simulink model "virtual_world_without_car"  (R2015b)
settings: Solver=ode3  StartTime=5  StopTime=simulationStop  FixedStep=0.04  RelTol=1e-3
PostLoadFcn:
  | if ~exist('visionlib','file') sl3ddemo_callbacks('DelayedError', gcs, 'Missing Library', 'This example requires Computer Vision System Toolbox.'); end; load octavia_testlap
values from neighbouring files (symbols this model uses):
  rotation_matrix = R_z * R_y * R_x    [frames_acquisition.m]
  sampleTime = 0.04    [frames_acquisition.m]
libraries: vrlib x26, visionsinks x1
Description:
  | Vehicle Dynamics Visualization with Video Output
  | 
  | This model extends the vr_octavia example and shows how to use
  | video output from the VR Video Output block.
  | 
  | This model performs a few simple operations on the output video signal.
  | The Video Viewer display then shows the resulting video stream where
  | the image edges are detected.
  | 
  | This model requires the Computer Vision System Toolbox(TM) product.
  | 
  | Such model has been used to implement an educational platform for
  | simulating Unmanned Aerial Vehicles aimed to detect and track moving
  | objects
settings Model: ExtModeArmWhenConnect=off  Creator=Giuseppe Silano  LastModifiedBy=giuse
settings DataIOCC: SaveFormat=Array  SignalLoggingName=sigsOut
settings OptimizationCC: BooleanDataType=off  OptimizeBlockIOStorage=off  BufferReuse=off  GlobalBufferReuse=off  ExpressionFolding=off  ExpressionDepthLimit=2147483647  LocalBlockOutputs=off  InitFltsAndDblsToZero=on
settings DebuggingCC: UnderspecifiedInitializationDetection=Classic  MergeDetectMultiDrivingBlocksExec=none  CheckExecutionContextPreStartOutputMsg=on  CheckExecutionContextRuntimeOutputMsg=on  SignalResolutionControl=TryResolveAllWithWarning  MultiTaskDSMMsg=warning  MultiTaskCondExecSysMsg=none  FcnCallInpInsideContextMsg=UseLocalSettings  StateNameClashWarn=warning
settings HardwareCC: ProdBitPerPointer=32  ProdLargestAtomicFloat=None  ProdIntDivRoundTo=Undefined  ProdEndianess=Unspecified  ProdWordSize=32  ProdHWDeviceType=32-bit Generic
settings RTWCC: RetainRTWFile=on
settings GRTTargetCC: TargetFcnLib=ansi_tfl_tmw.mat  GeneratePreprocessorConditionals=Disable all  CombineOutputUpdateFcns=off  GRTInterface=on
settings ConfigComp: CovModelRefEnable=Off  CovSFcnEnable=off

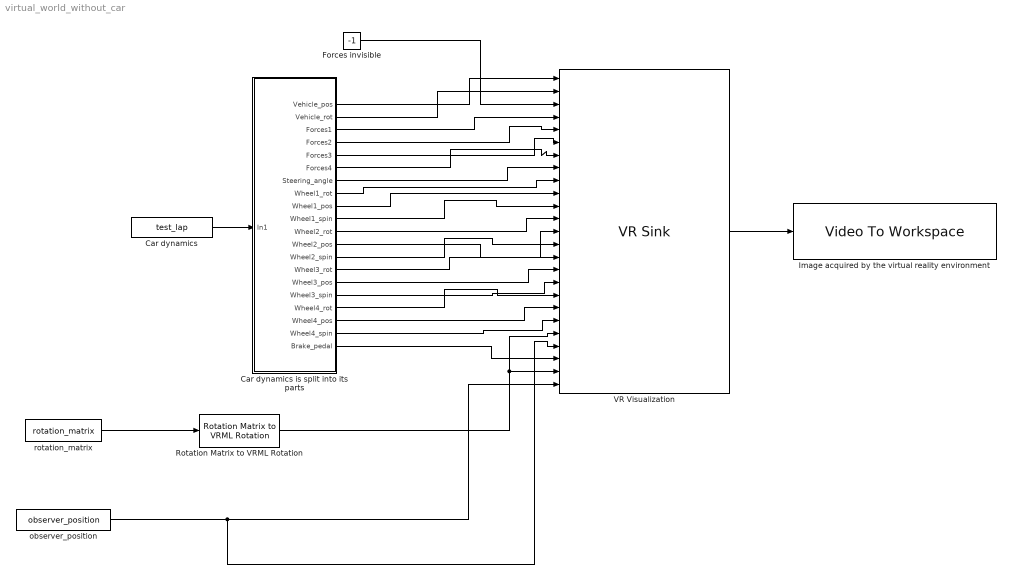
== system virtual_world_without_car ==
  Car dynamics : FromWorkspace  VariableName=test_lap  SampleTime=0.04  OutputAfterFinalValue=Holding final value
  "Car dynamics is split into its parts " : Subsystem
  Forces invisible : Constant  Value=-1
  Image acquired by the virtual reality environment : visionsinks/Video To Workspace  VariableName=image  NumInputs=1  DataLimit=1  DecimationFactor=1  LogFi=off  InPortLabels=R|G|B
  Rotation Matrix to VRML Rotation : vrlib/Utilities/Rotation Matrix to VRML Rotation  maxzero=1e-12
  VR Visualization : vrlib/VR Sink  InstantiateOnLoad=on  SampleTime=sampleTime  ViewEnable=on  RemoteChange=off  RemoteView=on  FieldsWritten=Vehicle_pos_Car1.translation.3.1.1.double#Vehicle_rot_Car1.rotation.4.1.1.double#Forces_visible_Car1.whichChoice.1.1.1.double#Force1_Car1.scale.3.1.1.double#Force2_Car1.scale.3.1.1.double#Force3_Car1.scale.3.1.1.double#Force4_Car1.scale.3.1.1.double#SteeringWheelAngle1_Car1.rotation.4.1.1.double#WheelFL_Car1.rotation.4.1.1.double#WheelFL_Car1.translation.3.1.1.double#WheelSpinFL_Car1.rotation.4.1.1.double#WheelFR_Car1.rotation.4.1.1.double#WheelFR_Car1.translation.3.1.1.double#WheelSpinFR_Car1.rotation.4.1.1.double#WheelRL_Car1.rotation.4.1.1.double#WheelRL_Car1.translation.3.1.1.double#WheelSpinRL_Car1.rotation.4.1.1.double#WheelRR_Car1.rotation.4.1.1.double#WheelRR_Car1.translation.3.1.1.double#WheelSpinRR_Car1.rotation.4.1.1.double#FlyingCamera.orientation.4.1.1.double#FlyingCamera.position.3.1.1.double#Brake_Switch_Car1.whichChoice.1.1.1.double#Osservatore_esterno:drone.orientation.4.1.1.double#Osservatore_esterno:drone.position.3.1.1.double  WorldFileName=octavia_scene.wrl  WorldDescription=Vehicle dynamics visualization  AutoView=on  VideoDimensions=[800 600]  AllowVariableSize=off  FigureProperties="{'Position', 'Name', 'Viewpoint', 'CameraBound', 'CameraDirection', 'CameraPosition', 'CameraUpVector', 'ZoomFactor', 'Antialiasing', 'Headlight', 'Lighting', 'NavPanel', 'Sound', 'StatusBar', 'Stereo3D', 'Stereo3DCameraOffset', 'Stereo3DHIT', 'ToolBar', 'Textures', 'Transparency', 'Triad', 'Wireframe', 'NavZones', 'NavMode', 'NavSpeed', 'CaptureFileFormat', 'CaptureFileName', 'Record2DCompressMethod', 'Record2DCompressQuality', 'Record2D', 'Record2DFileName', 'Record2DFPS'; [5.0000000000000000e+00   9.2000000000000000e+01   5.7600000000000000e+02   3.8000000000000000e+02], 'Vehicle dynamics visualization', 'Car - View from Right Above Ahead', 'on', [0.0000000000000000e+00   0.0000000000000000e+00  -1.0000000000000000e+00], [0.0000000000000000e+00   0.0000000000000000e+00   0.0000000000000000e+00], [0.0000000000000000e+00   1.0000000000000000e+00   0.0000000000000000e+00], [1.0000000000000000e+00], 'on', 'off', 'on', 'halfbar', 'on', 'on', 'off', [1.0000000149011612e-01], [0.0000000000000000e+00], 'on', 'on', 'on', 'none', 'off', 'off', 'walk', 'normal', 'tif', '%f_anim_%n.tif', 'auto', [7.5000000000000000e+01], 'off', '%f_anim_%n.avi', 'auto'; [5.8600000000000000e+02   6.0000000000000000e+01   6.0000000000000000e+02   8.0000000000000000e+02], 'Vehicle dynamics visualization', 'Osservatore_esterno:drone', 'on', [0.0000000000000000e+00   0.0000000000000000e+00  -1.0000000000000000e+00], [0.0000000000000000e+00   0.0000000000000000e+00   0.0000000000000000e+00], [0.0000000000000000e+00   1.0000000000000000e+00   0.0000000000000000e+00], [1.0000000000000000e+00], 'on', 'off', 'on', 'none', 'on', 'off', 'off', [1.0000000149011612e-01], [0.0000000000000000e+00], 'off', 'on', 'on', 'none', 'off', 'off', 'walk', 'normal', 'tif', '%f_anim_%n.tif', 'auto', [7.5000000000000000e+01], 'off', '***video***', [1.5000000000000000e+01]}"
  observer_position : FromWorkspace  VariableName=observer_position  SampleTime=0
  rotation_matrix : Constant  Value=rotation_matrix
  wires:
  Car dynamics/1 -> "Car dynamics is split into its parts "/1(In1)
  VR Visualization/1 -> Image acquired by the virtual reality environment/1
  "Car dynamics is split into its parts "/1(Vehicle_pos) -> VR Visualization/1
  "Car dynamics is split into its parts "/2(Vehicle_rot) -> VR Visualization/2
  Forces invisible/1 -> VR Visualization/3
  "Car dynamics is split into its parts "/3(Forces1) -> VR Visualization/4
  "Car dynamics is split into its parts "/4(Forces2) -> VR Visualization/5
  "Car dynamics is split into its parts "/5(Forces3) -> VR Visualization/6
  "Car dynamics is split into its parts "/6(Forces4) -> VR Visualization/7
  "Car dynamics is split into its parts "/7(Steering_angle) -> VR Visualization/8
  "Car dynamics is split into its parts "/8(Wheel1_rot) -> VR Visualization/9
  "Car dynamics is split into its parts "/9(Wheel1_pos) -> VR Visualization/10
  "Car dynamics is split into its parts "/10(Wheel1_spin) -> VR Visualization/11
  "Car dynamics is split into its parts "/11(Wheel2_rot) -> VR Visualization/12
  "Car dynamics is split into its parts "/12(Wheel2_pos) -> VR Visualization/13
  "Car dynamics is split into its parts "/13(Wheel2_spin) -> VR Visualization/14
  "Car dynamics is split into its parts "/14(Wheel3_rot) -> VR Visualization/15
  "Car dynamics is split into its parts "/15(Wheel3_pos) -> VR Visualization/16
  "Car dynamics is split into its parts "/16(Wheel3_spin) -> VR Visualization/17
  "Car dynamics is split into its parts "/17(Wheel4_rot) -> VR Visualization/18
  "Car dynamics is split into its parts "/18(Wheel4_pos) -> VR Visualization/19
  "Car dynamics is split into its parts "/19(Wheel4_spin) -> VR Visualization/20
  observer_position/1 -> VR Visualization/22, VR Visualization/25
  "Car dynamics is split into its parts "/20(Brake_pedal) -> VR Visualization/23
  Rotation Matrix to VRML Rotation/1 -> VR Visualization/21, VR Visualization/24
  rotation_matrix/1 -> Rotation Matrix to VRML Rotation/1

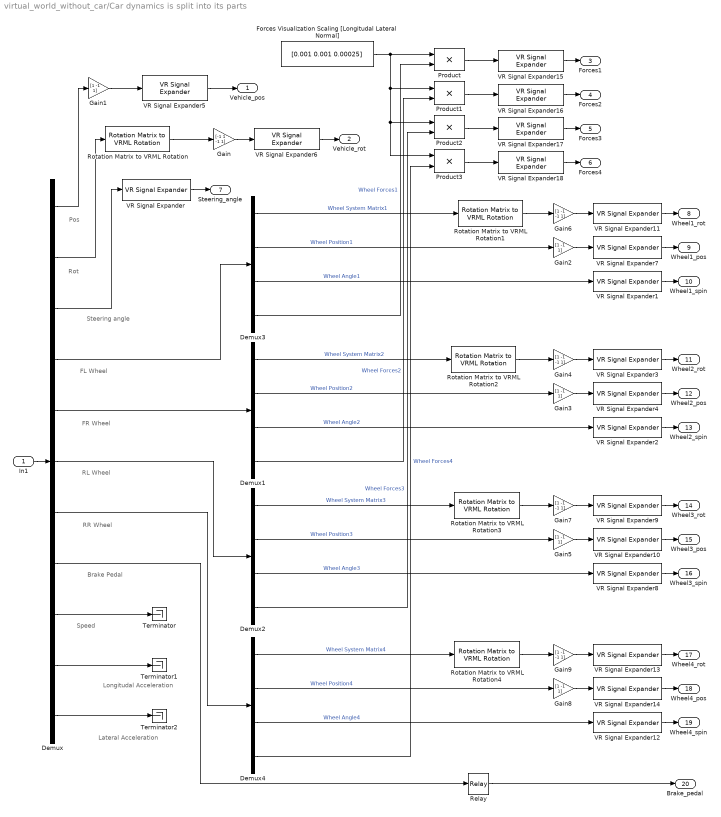
== system virtual_world_without_car/Car dynamics is split into its parts  ==
  note: Steering angle
  note: FL Wheel
  note: FR Wheel
  note: RL Wheel
  note: RR Wheel
  note: Brake Pedal
  note: Pos
  note: Rot
  note: Speed
  note: Longitudal Acceleration
  note: Lateral Acceleration
  In1 : Inport
  Demux : Demux  Outputs=[3,9,1,16,16,16,16,1,1,1,1]
  Demux{1..4} (4 alike) : Demux  Outputs=[9,3,1,3]
  Forces Visualization Scaling [Longitudal Lateral Normal] : Constant  Value=[0.001 0.001 0.00025]
  Gain : Gain  Gain=[-1 1 -1 1]  SaturateOnIntegerOverflow=on  OutDataTypeStr=Inherit: Same as input  ParamDataTypeStr=Inherit: Same as input
  Gain{1..3,5,8} (5 alike) : Gain  Gain=[1 -1 1]  SaturateOnIntegerOverflow=on  OutDataTypeStr=Inherit: Same as input  ParamDataTypeStr=Inherit: Same as input
  Gain{4,6..7,9} (4 alike) : Gain  Gain=[1 -1 -1 1]  SaturateOnIntegerOverflow=on  OutDataTypeStr=Inherit: Same as input  ParamDataTypeStr=Inherit: Same as input
  Product{,1..3} (4 alike) : Product  SaturateOnIntegerOverflow=on  OutDataTypeStr=Inherit: Same as first input
  Relay : Relay
  Rotation Matrix to VRML Rotation{,1..4} (5 alike) : vrlib/Utilities/Rotation Matrix to VRML Rotation  maxzero=1e-12
  Terminator : Terminator
  Terminator1 : Terminator
  Terminator2 : Terminator
  VR Signal Expander{,1..2,8,12} (5 alike) : vrlib/VR Signal Expander  outwidth=4  outidx=[4]
  VR Signal Expander{4,7,10,14} (4 alike) : vrlib/VR Signal Expander  outwidth=3  outidx=[1 3 2 ]
  VR Signal Expander{3,6,9,11,13} (5 alike) : vrlib/VR Signal Expander  outwidth=4  outidx=[1 3 2 4]
  VR Signal Expander{5,15..18} (5 alike) : vrlib/VR Signal Expander  outwidth=3  outidx=[1 3 2]
  Vehicle_pos : Outport
  Vehicle_rot : Outport  Port=2
  Forces1 : Outport  Port=3
  Forces2 : Outport  Port=4
  Forces3 : Outport  Port=5
  Forces4 : Outport  Port=6
  Steering_angle : Outport  Port=7
  Wheel1_rot : Outport  Port=8
  Wheel1_pos : Outport  Port=9
  Wheel1_spin : Outport  Port=10
  Wheel2_rot : Outport  Port=11
  Wheel2_pos : Outport  Port=12
  Wheel2_spin : Outport  Port=13
  Wheel3_rot : Outport  Port=14
  Wheel3_pos : Outport  Port=15
  Wheel3_spin : Outport  Port=16
  Wheel4_rot : Outport  Port=17
  Wheel4_pos : Outport  Port=18
  Wheel4_spin : Outport  Port=19
  Brake_pedal : Outport  Port=20
  wires:
  Gain1/1 -> VR Signal Expander5/1
  Rotation Matrix to VRML Rotation/1 -> Gain/1
  Gain/1 -> VR Signal Expander6/1
  Gain6/1 -> VR Signal Expander11/1
  Gain2/1 -> VR Signal Expander7/1
  Demux3/1 -> Rotation Matrix to VRML Rotation1/1  "Wheel System Matrix1"
  Demux3/2 -> Gain2/1  "Wheel Position1"
  Demux3/3 -> VR Signal Expander1/1  "Wheel Angle1"
  Gain4/1 -> VR Signal Expander3/1
  Rotation Matrix to VRML Rotation2/1 -> Gain4/1
  Gain3/1 -> VR Signal Expander4/1
  Demux1/1 -> Rotation Matrix to VRML Rotation2/1  "Wheel System Matrix2"
  Demux1/2 -> Gain3/1  "Wheel Position2"
  Demux1/3 -> VR Signal Expander2/1  "Wheel Angle2"
  Gain7/1 -> VR Signal Expander9/1
  Rotation Matrix to VRML Rotation3/1 -> Gain7/1
  Demux2/4 -> Product2/2  "Wheel Forces3"
  Gain5/1 -> VR Signal Expander10/1
  Demux2/1 -> Rotation Matrix to VRML Rotation3/1  "Wheel System Matrix3"
  Demux2/2 -> Gain5/1  "Wheel Position3"
  Demux2/3 -> VR Signal Expander8/1  "Wheel Angle3"
  Gain9/1 -> VR Signal Expander13/1
  Rotation Matrix to VRML Rotation4/1 -> Gain9/1
  Demux4/4 -> Product3/2  "Wheel Forces4"
  Gain8/1 -> VR Signal Expander14/1
  Demux4/1 -> Rotation Matrix to VRML Rotation4/1  "Wheel System Matrix4"
  Demux4/2 -> Gain8/1  "Wheel Position4"
  Demux4/3 -> VR Signal Expander12/1  "Wheel Angle4"
  VR Signal Expander5/1 -> Vehicle_pos/1
  Demux3/4 -> Product/2  "Wheel Forces1"
  Demux1/4 -> Product1/2  "Wheel Forces2"
  Product/1 -> VR Signal Expander15/1
  Product1/1 -> VR Signal Expander16/1
  Product2/1 -> VR Signal Expander17/1
  Product3/1 -> VR Signal Expander18/1
  VR Signal Expander6/1 -> Vehicle_rot/1
  VR Signal Expander15/1 -> Forces1/1
  VR Signal Expander16/1 -> Forces2/1
  VR Signal Expander17/1 -> Forces3/1
  VR Signal Expander18/1 -> Forces4/1
  VR Signal Expander/1 -> Steering_angle/1
  VR Signal Expander11/1 -> Wheel1_rot/1
  In1/1 -> Demux/1
  VR Signal Expander7/1 -> Wheel1_pos/1
  VR Signal Expander1/1 -> Wheel1_spin/1
  VR Signal Expander3/1 -> Wheel2_rot/1
  VR Signal Expander4/1 -> Wheel2_pos/1
  VR Signal Expander2/1 -> Wheel2_spin/1
  VR Signal Expander9/1 -> Wheel3_rot/1
  VR Signal Expander10/1 -> Wheel3_pos/1
  VR Signal Expander8/1 -> Wheel3_spin/1
  VR Signal Expander13/1 -> Wheel4_rot/1
  VR Signal Expander14/1 -> Wheel4_pos/1
  VR Signal Expander12/1 -> Wheel4_spin/1
  Demux/8 -> Relay/1
  Relay/1 -> Brake_pedal/1
  Demux/1 -> Gain1/1
  Demux/2 -> Rotation Matrix to VRML Rotation/1
  Demux/3 -> VR Signal Expander/1
  Demux/4 -> Demux3/1
  Demux/5 -> Demux1/1
  Demux/6 -> Demux2/1
  Demux/7 -> Demux4/1
  Forces Visualization Scaling [Longitudal Lateral Normal]/1 -> Product/1, Product1/1, Product2/1, Product3/1
  Rotation Matrix to VRML Rotation1/1 -> Gain6/1
  Demux/9 -> Terminator/1
  Demux/10 -> Terminator1/1
  Demux/11 -> Terminator2/1
